simulink model "Attitude"  (R2023b)
settings: Solver=VariableStepAuto  StartTime=0.0  StopTime=10.0  RelTol=1e-3
libraries: simulink_extras x6, aerolibutil x6, vrlib x4, simulink x4, sharedtransform x3, dspindex x3
settings Model: Creator=Saif Mohamed  LastModifiedBy=saifg

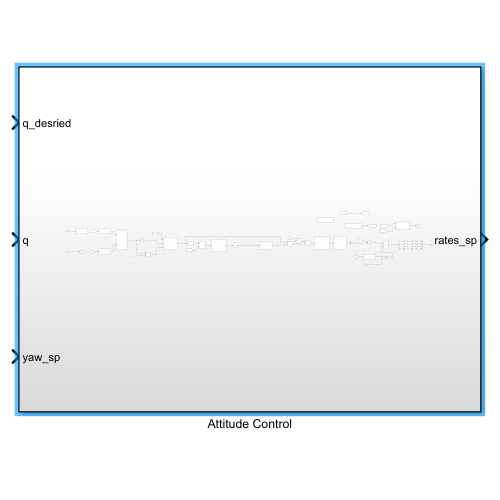
[thumbnail: Simulink's stored preview of the top-level diagram]
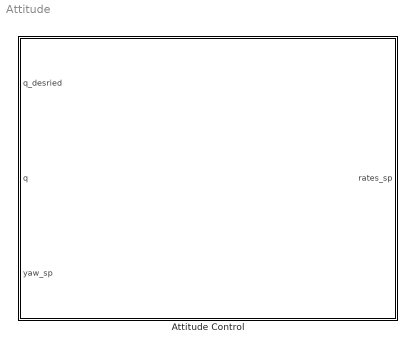
== system Attitude ==
  Attitude Control : Subsystem

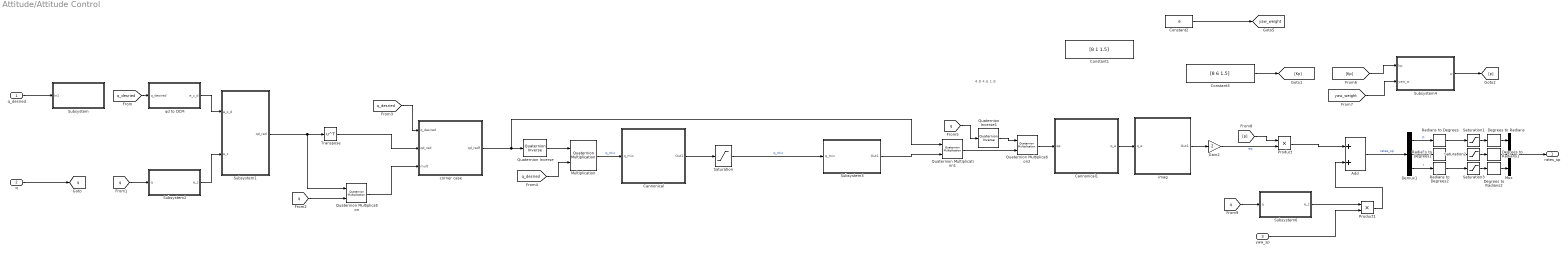
== system Attitude/Attitude Control ==
  note: 4.8 4.6 1.8
  q_desried : Inport
  q : Inport  Port=2
  yaw_sp : Inport  Port=3
  Add : Sum
  Cannonical : Subsystem
  Cannonical1 : Subsystem
  Constant1 : Constant  Value=[8 1 1.5]
  Constant2 : Constant  Value=.6
  Constant3 : Constant  Value=[8 6 1.5]
  Degrees to Radians : simulink_extras/Transformations/Degrees to Radians
  Degrees to Radians1 : simulink_extras/Transformations/Degrees to Radians
  Degrees to Radians2 : simulink_extras/Transformations/Degrees to Radians
  Demux1 : Demux  Outputs=3
  Gain2 : Gain  Gain=2
  Multiplication : aerolibutil/Quaternion Multiplication
  Mux : Mux  Inputs=3
  Product : Product
  Product1 : Product
  Quaternion Inverse : aerolibutil/Quaternion Inverse
  Quaternion Inverse1 : aerolibutil/Quaternion Inverse
  Quaternion Multiplication : aerolibutil/Quaternion Multiplication
  Quaternion Multiplication1 : aerolibutil/Quaternion Multiplication
  Quaternion Multiplication2 : aerolibutil/Quaternion Multiplication
  Radians to Degrees : simulink_extras/Transformations/Radians to Degrees
  Radians to Degrees1 : simulink_extras/Transformations/Radians to Degrees
  Radians to Degrees2 : simulink_extras/Transformations/Radians to Degrees
  Saturation : Saturate  UpperLimit=1  LowerLimit=-1
  Saturation1 : Saturate  UpperLimit=220  LowerLimit=-220
  Saturation2 : Saturate  UpperLimit=220  LowerLimit=-220
  Saturation3 : Saturate  UpperLimit=200  LowerLimit=-200
  Subsystem : Subsystem
  Subsystem1 : Subsystem
  Subsystem2 : Subsystem
  Subsystem3 : Subsystem
  Subsystem4 : Subsystem
  Subsystem6 : Subsystem
  Transpose : Math  Operator=transpose
  corner case : Subsystem
  imag : Subsystem
  qd to DCM : Subsystem
  rates_sp : Outport
  tag scope: q=global, yaw_weight=global
  wires:
  q_desried/1 -> Subsystem/1(In1)
  q/1 -> [q]
  [q_desried] -> qd to DCM/1(q_desired)
  [q] -> Subsystem2/1(q)
  qd to DCM/1(e_z_d) -> Subsystem1/1(e_z_d)
  Subsystem2/1(e_z) -> Subsystem1/2(e_z)
  Subsystem1/1(qd_red) -> Transpose/1, Quaternion Multiplication/1
  [q] -> Quaternion Multiplication/2
  Transpose/1 -> corner case/2(qd_red)
  Quaternion Multiplication/1 -> corner case/3(mult)
  [q_desried] -> corner case/1(q_desired)
  Quaternion Inverse/1 -> Multiplication/1
  [q_desried] -> Multiplication/2
  Multiplication/1 -> Cannonical/1("q_mix ")  "q_mix"
  Cannonical/1(Out1) -> Saturation/1
  Constant2/1 -> [yaw_weight]
  Saturation/1 -> Subsystem3/1(q_mix)  "q_mix"
  Subsystem3/1(Out1) -> Quaternion Multiplication1/2
  Quaternion Multiplication1/1 -> Quaternion Multiplication2/2
  Quaternion Inverse1/1 -> Quaternion Multiplication2/1
  [q] -> Quaternion Inverse1/1
  Quaternion Multiplication2/1 -> Cannonical1/1("qe ")
  Cannonical1/1(q_e) -> imag/1(q_e)
  imag/1(Out1) -> Gain2/1
  Gain2/1 -> Product/2  "eq"
  Constant3/1 -> [Kp]
  [Kp] -> Subsystem4/1(kp)
  [yaw_weight] -> Subsystem4/2(yaw_w)
  Subsystem4/1(p) -> [p]
  [p] -> Product/1
  Product/1 -> Add/1
  [q] -> Subsystem6/1(q)
  Subsystem6/1(e_z) -> Product1/1
  yaw_sp/1 -> Product1/2
  Product1/1 -> Add/2
  Add/1 -> Demux1/1  "rates_sp"
  Demux1/1 -> Radians to Degrees/1  "p"
  Demux1/2 -> Radians to Degrees1/1  "q"
  Demux1/3 -> Radians to Degrees2/1  "r"
  Radians to Degrees/1 -> Saturation1/1
  Radians to Degrees1/1 -> Saturation2/1
  Radians to Degrees2/1 -> Saturation3/1
  Saturation1/1 -> Degrees to Radians/1
  Saturation2/1 -> Degrees to Radians1/1
  Saturation3/1 -> Degrees to Radians2/1
  Mux/1 -> rates_sp/1
  Degrees to Radians/1 -> Mux/1
  Degrees to Radians1/1 -> Mux/2
  Degrees to Radians2/1 -> Mux/3
  corner case/1(qd_redf) -> Quaternion Multiplication1/1, Quaternion Inverse/1

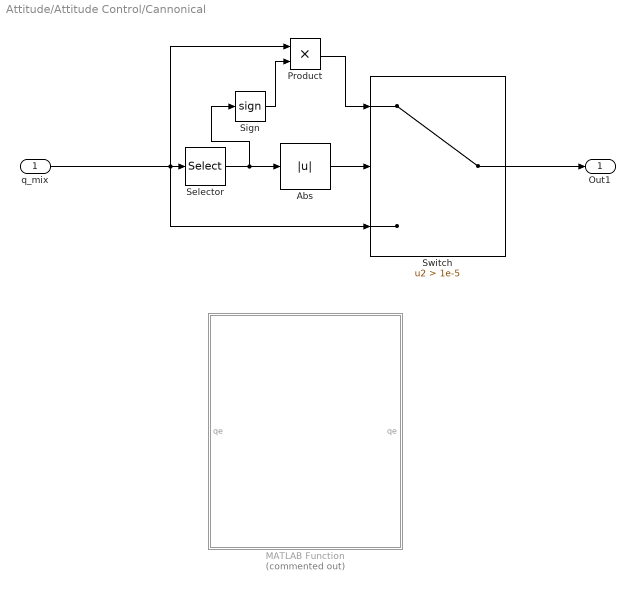
== system Attitude/Attitude Control/Cannonical ==
  "q_mix " : Inport
  Abs : Abs  SaturateOnIntegerOverflow=off
  MATLAB Function : MATLAB Function  Commented=on  TreatAsAtomicUnit=on
  Product : Product
  Selector : Selector  InputPortWidth=4  IndexOptions=Index vector (dialog)  Indices=[1]  OutputSizes=1
  Sign : Signum
  Switch : Switch  Criteria=u2 > Threshold  Threshold=1e-5  SaturateOnIntegerOverflow=off  InputSameDT=off
  Out1 : Outport
  wires:
  "q_mix "/1 -> Product/1, Selector/1, Switch/3
  Selector/1 -> Sign/1, Abs/1
  Abs/1 -> Switch/2
  Switch/1 -> Out1/1
  Product/1 -> Switch/1
  Sign/1 -> Product/2

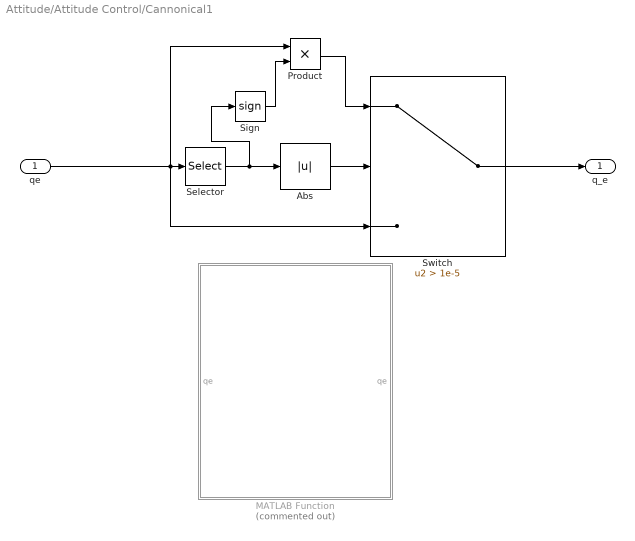
== system Attitude/Attitude Control/Cannonical1 ==
  "qe " : Inport
  Abs : Abs  SaturateOnIntegerOverflow=off
  MATLAB Function : MATLAB Function  Commented=on  TreatAsAtomicUnit=on
  Product : Product
  Selector : Selector  InputPortWidth=4  IndexOptions=Index vector (dialog)  Indices=[1]  OutputSizes=1
  Sign : Signum
  Switch : Switch  Criteria=u2 > Threshold  Threshold=1e-5  SaturateOnIntegerOverflow=off  InputSameDT=off
  q_e : Outport
  wires:
  "qe "/1 -> Product/1, Selector/1, Switch/3
  Selector/1 -> Sign/1, Abs/1
  Abs/1 -> Switch/2
  Switch/1 -> q_e/1
  Product/1 -> Switch/1
  Sign/1 -> Product/2

== system Attitude/Attitude Control/Subsystem ==
  In1 : Inport
  Normalize Vector : vrlib/Utilities/Normalize Vector  maxzero=0
  tag scope: q_desried=global
  wires:
  Normalize Vector/1 -> [q_desried]
  In1/1 -> Normalize Vector/1

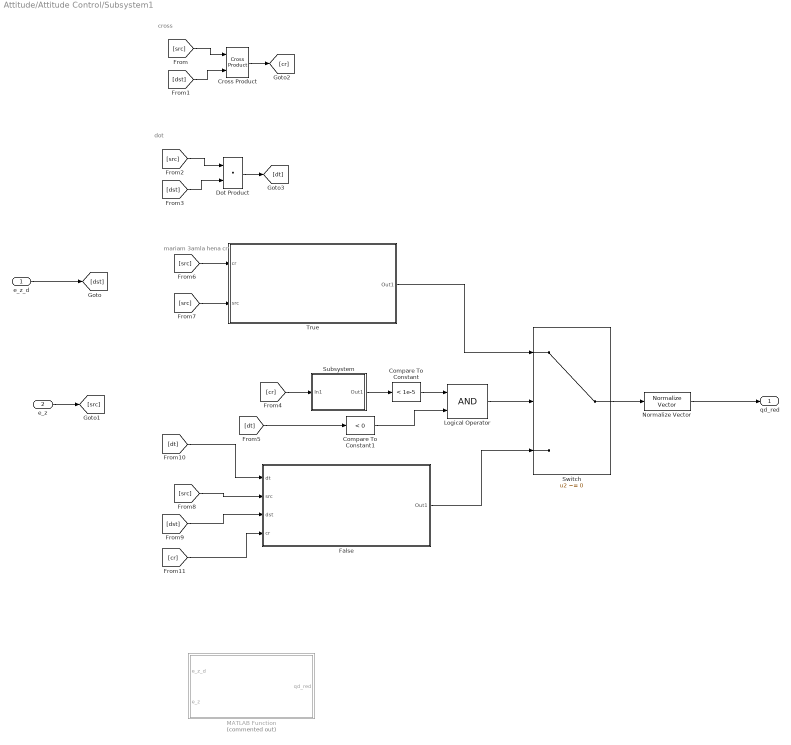
== system Attitude/Attitude Control/Subsystem1 ==
  note: mariam 3amla hena cr
  note: cross
  note: dot
  e_z_d : Inport
  e_z : Inport  Port=2
  Compare To Constant : simulink/Logic and Bit Operations/Compare To Constant  relop=<  const=1e-5  OutDataTypeStr=boolean
  Compare To Constant1 : simulink/Logic and Bit Operations/Compare To Constant  relop=<  const=0  OutDataTypeStr=boolean
  Cross Product : vrlib/Utilities/Cross Product
  Dot Product : DotProduct  OutDataTypeStr=Inherit: Inherit via internal rule
  False : Subsystem
  Logical Operator : Logic  AllPortsSameDT=off  OutDataTypeStr=boolean
  MATLAB Function : MATLAB Function  Commented=on  TreatAsAtomicUnit=on
  Normalize Vector : vrlib/Utilities/Normalize Vector  maxzero=0
  Subsystem : Subsystem
  Switch : Switch  Criteria=u2 ~= 0  SaturateOnIntegerOverflow=off  InputSameDT=off
  True : Subsystem
  qd_red : Outport
  wires:
  e_z_d/1 -> [dst]
  e_z/1 -> [src]
  [src] -> Cross Product/1
  [dst] -> Cross Product/2
  Cross Product/1 -> [cr]
  [src] -> Dot Product/1
  [dst] -> Dot Product/2
  Dot Product/1 -> [dt]
  [cr] -> Subsystem/1(In1)
  Subsystem/1(Out1) -> Compare To Constant/1
  Compare To Constant/1 -> Logical Operator/1
  [dt] -> Compare To Constant1/1
  Compare To Constant1/1 -> Logical Operator/2
  Logical Operator/1 -> Switch/2
  [src] -> True/1(cr)
  [src] -> True/2(src)
  True/1(Out1) -> Switch/1
  [src] -> False/2(src)
  [dst] -> False/3(dst)
  [dt] -> False/1(dt)
  [cr] -> False/4(cr)
  False/1(Out1) -> Switch/3
  Switch/1 -> Normalize Vector/1
  Normalize Vector/1 -> qd_red/1

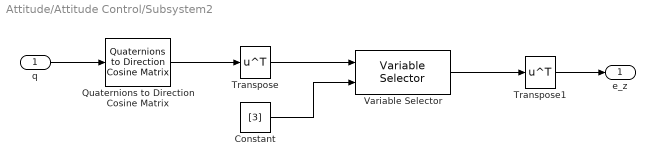
== system Attitude/Attitude Control/Subsystem2 ==
  q : Inport
  Constant : Constant  Value=[3]
  Quaternions to Direction Cosine Matrix : sharedtransform/Quaternions to  Direction Cosine Matrix  aMode=aMode
      settings: LibrarySourceBlock=|
      | aerolibtransform2/Quaternions to
      | Direction Cosine Matrix
  Transpose : Math  Operator=transpose
  Transpose1 : Math  Operator=transpose
  Variable Selector : dspindex/Variable Selector  NumInputs=1  rowsOrCols=Columns  IdxMode=Variable  Elements=[1 3]  ZerOneIdxMode=One-based  errmode=Clip Index  FillMode=on  FillValues=0
  e_z : Outport
  wires:
  Transpose1/1 -> e_z/1
  Variable Selector/1 -> Transpose1/1
  Constant/1 -> Variable Selector/2
  Transpose/1 -> Variable Selector/1
  Quaternions to Direction Cosine Matrix/1 -> Transpose/1
  q/1 -> Quaternions to Direction Cosine Matrix/1

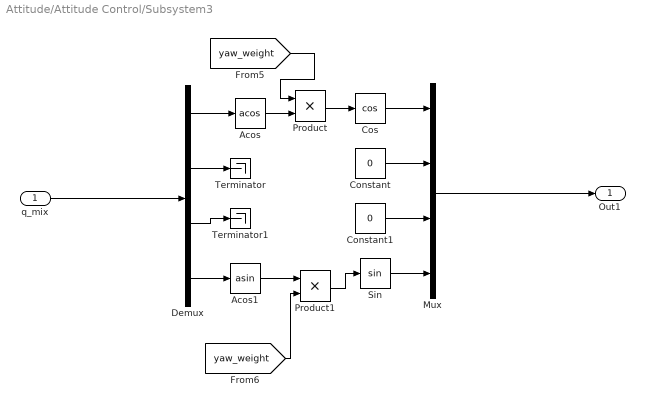
== system Attitude/Attitude Control/Subsystem3 ==
  q_mix : Inport
  Acos : Trigonometry  Operator=acos
  Acos1 : Trigonometry  Operator=asin
  Constant : Constant  Value=0
  Constant1 : Constant  Value=0
  Cos : Trigonometry  Operator=cos
  Demux : Demux
  Mux : Mux
  Product : Product
  Product1 : Product
  Sin : Trigonometry
  Terminator : Terminator
  Terminator1 : Terminator
  Out1 : Outport
  wires:
  Sin/1 -> Mux/4
  Acos/1 -> Product/2
  [yaw_weight] -> Product/1
  Product/1 -> Cos/1
  q_mix/1 -> Demux/1
  Demux/4 -> Acos1/1
  Product1/1 -> Sin/1
  Demux/1 -> Acos/1
  Cos/1 -> Mux/1
  Mux/1 -> Out1/1
  Acos1/1 -> Product1/1
  [yaw_weight] -> Product1/2
  Demux/2 -> Terminator/1
  Demux/3 -> Terminator1/1
  Constant1/1 -> Mux/3
  Constant/1 -> Mux/2

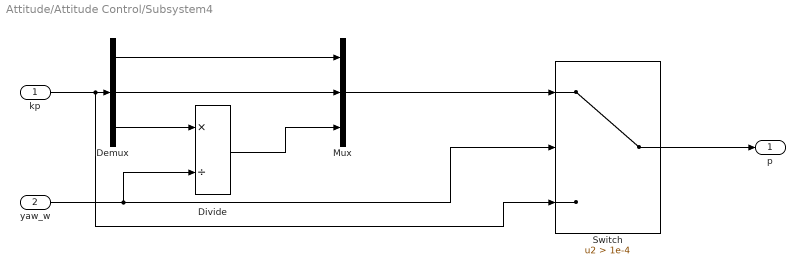
== system Attitude/Attitude Control/Subsystem4 ==
  kp : Inport
  yaw_w : Inport  Port=2
  Demux : Demux  Outputs=3
  Divide : Product  Inputs=*/
  Mux : Mux  Inputs=3
  Switch : Switch  Criteria=u2 > Threshold  Threshold=1e-4  SaturateOnIntegerOverflow=off  InputSameDT=off
  p : Outport
  wires:
  yaw_w/1 -> Switch/2, Divide/2
  Mux/1 -> Switch/1
  kp/1 -> Switch/3, Demux/1
  Demux/1 -> Mux/1
  Demux/2 -> Mux/2
  Demux/3 -> Divide/1
  Divide/1 -> Mux/3
  Switch/1 -> p/1

== system Attitude/Attitude Control/Subsystem6 ==
  q : Inport
  Constant : Constant  Value=[3]
  Quaternions to Direction Cosine Matrix : sharedtransform/Quaternions to  Direction Cosine Matrix  aMode=aMode
      settings: LibrarySourceBlock=|
      | aerolibtransform2/Quaternions to
      | Direction Cosine Matrix
  Transpose : Math  Operator=transpose
  Variable Selector : dspindex/Variable Selector  NumInputs=1  rowsOrCols=Columns  IdxMode=Variable  Elements=[1 3]  ZerOneIdxMode=One-based  errmode=Clip Index  FillMode=on  FillValues=0
  e_z : Outport
  wires:
  Variable Selector/1 -> e_z/1
  Constant/1 -> Variable Selector/2
  Transpose/1 -> Variable Selector/1
  Quaternions to Direction Cosine Matrix/1 -> Transpose/1
  q/1 -> Quaternions to Direction Cosine Matrix/1

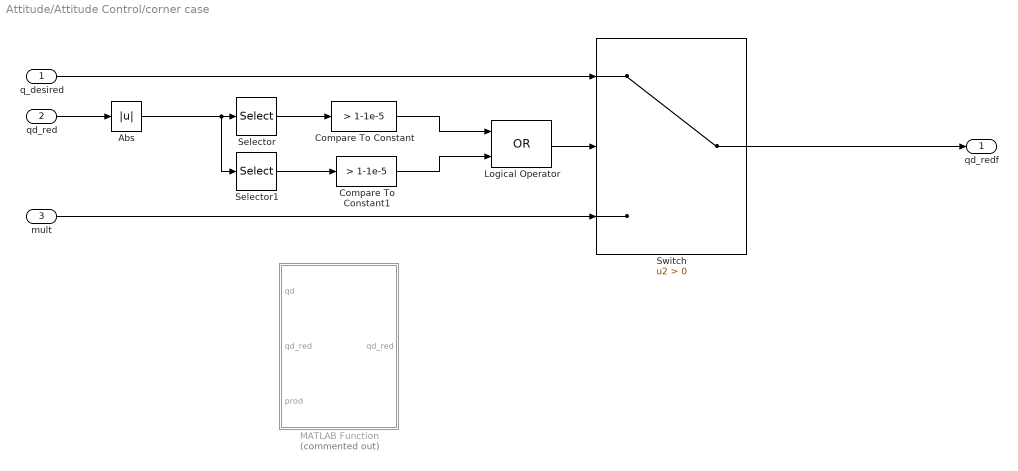
== system Attitude/Attitude Control/corner case ==
  q_desired : Inport
  qd_red : Inport  Port=2
  mult : Inport  Port=3
  Abs : Abs  SaturateOnIntegerOverflow=off
  Compare To Constant : simulink/Logic and Bit Operations/Compare To Constant  relop=>  const=1-1e-5  OutDataTypeStr=boolean
  Compare To Constant1 : simulink/Logic and Bit Operations/Compare To Constant  relop=>  const=1-1e-5  OutDataTypeStr=boolean
  Logical Operator : Logic  Operator=OR  AllPortsSameDT=off  OutDataTypeStr=boolean
  MATLAB Function : MATLAB Function  Commented=on  TreatAsAtomicUnit=on
  Selector : Selector  InputPortWidth=4  IndexOptions=Index vector (dialog)  Indices=[2]  OutputSizes=1
  Selector1 : Selector  InputPortWidth=4  IndexOptions=Index vector (dialog)  Indices=[3]  OutputSizes=1
  Switch : Switch  Criteria=u2 > Threshold  SaturateOnIntegerOverflow=off  InputSameDT=off
  qd_redf : Outport
  wires:
  Abs/1 -> Selector1/1, Selector/1
  Selector/1 -> Compare To Constant/1
  Selector1/1 -> Compare To Constant1/1
  Compare To Constant/1 -> Logical Operator/1
  Compare To Constant1/1 -> Logical Operator/2
  Switch/1 -> qd_redf/1
  Logical Operator/1 -> Switch/2
  q_desired/1 -> Switch/1
  mult/1 -> Switch/3
  qd_red/1 -> Abs/1

== system Attitude/Attitude Control/imag ==
  q_e : Inport
  Demux : Demux
  Mux : Mux  Inputs=3
  Terminator : Terminator
  Out1 : Outport
  wires:
  Mux/1 -> Out1/1
  q_e/1 -> Demux/1
  Demux/1 -> Terminator/1
  Demux/2 -> Mux/1
  Demux/3 -> Mux/2
  Demux/4 -> Mux/3

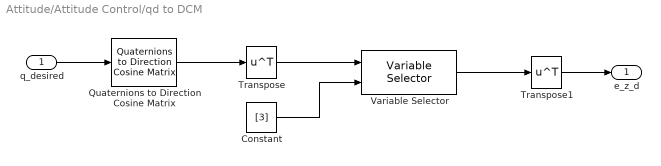
== system Attitude/Attitude Control/qd to DCM ==
  q_desired : Inport
  Constant : Constant  Value=[3]
  Quaternions to Direction Cosine Matrix : sharedtransform/Quaternions to  Direction Cosine Matrix  aMode=aMode
      settings: LibrarySourceBlock=|
      | aerolibtransform2/Quaternions to
      | Direction Cosine Matrix
  Transpose : Math  Operator=transpose
  Transpose1 : Math  Operator=transpose
  Variable Selector : dspindex/Variable Selector  NumInputs=1  rowsOrCols=Columns  IdxMode=Variable  Elements=[1 3]  ZerOneIdxMode=One-based  errmode=Clip Index  FillMode=on  FillValues=0
  e_z_d : Outport
  wires:
  q_desired/1 -> Quaternions to Direction Cosine Matrix/1
  Quaternions to Direction Cosine Matrix/1 -> Transpose/1
  Transpose/1 -> Variable Selector/1
  Constant/1 -> Variable Selector/2
  Variable Selector/1 -> Transpose1/1
  Transpose1/1 -> e_z_d/1

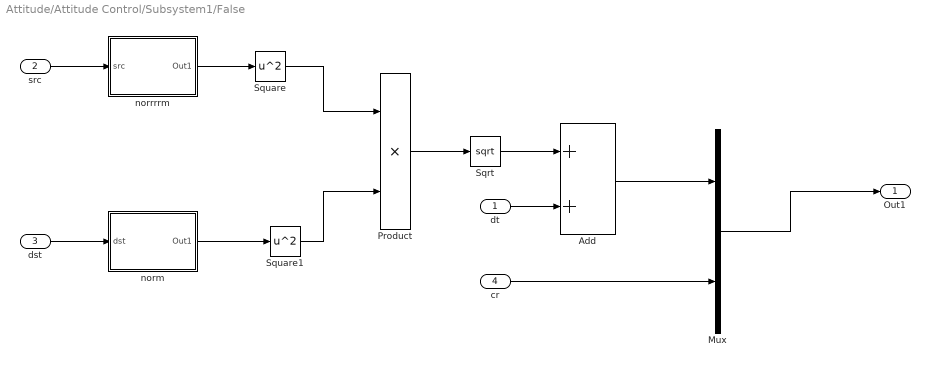
== system Attitude/Attitude Control/Subsystem1/False ==
  dt : Inport
  src : Inport  Port=2
  dst : Inport  Port=3
  cr : Inport  Port=4
  Add : Sum
  Mux : Mux  Inputs=2
  Product : Product
  Sqrt : Sqrt
  Square : Math  Operator=square
  Square1 : Math  Operator=square
  norm : Subsystem
  norrrrm : Subsystem
  Out1 : Outport
  wires:
  src/1 -> norrrrm/1(src)
  dst/1 -> norm/1(dst)
  norrrrm/1(Out1) -> Square/1
  norm/1(Out1) -> Square1/1
  Square/1 -> Product/1
  Square1/1 -> Product/2
  Product/1 -> Sqrt/1
  Sqrt/1 -> Add/1
  dt/1 -> Add/2
  Add/1 -> Mux/1
  Mux/1 -> Out1/1
  cr/1 -> Mux/2

== system Attitude/Attitude Control/Subsystem1/Subsystem ==
  In1 : Inport
  Square : Math  Operator=square
  Square1 : Math  Operator=square
  Sum of Elements : Sum  Inputs=+
  Out1 : Outport
  wires:
  In1/1 -> Square/1
  Square/1 -> Sum of Elements/1
  Sum of Elements/1 -> Square1/1
  Square1/1 -> Out1/1

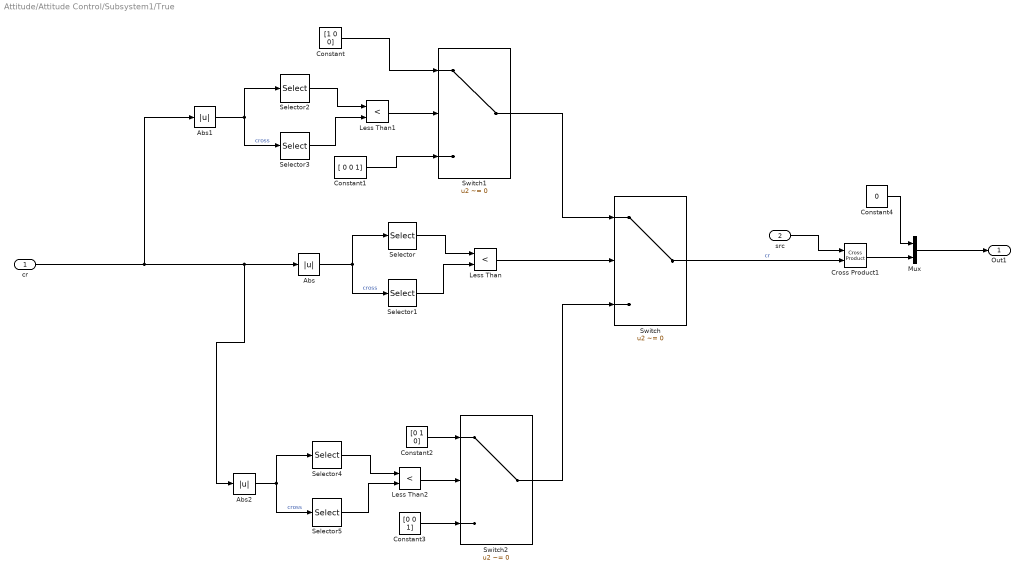
== system Attitude/Attitude Control/Subsystem1/True ==
  cr : Inport
  src : Inport  Port=2
  Abs : Abs  SaturateOnIntegerOverflow=off
  Abs1 : Abs  SaturateOnIntegerOverflow=off
  Abs2 : Abs  SaturateOnIntegerOverflow=off
  Constant : Constant  Value=[1 0 0]
  Constant1 : Constant  Value=[ 0 0 1]
  Constant2 : Constant  Value=[0 1 0]
  Constant3 : Constant  Value=[0 0 1]
  Constant4 : Constant  Value=0
  Cross Product1 : vrlib/Utilities/Cross Product
  Less Than : RelationalOperator  Operator=<  OutDataTypeStr=boolean  RndMeth=Simplest  InputSameDT=off
  Less Than1 : RelationalOperator  Operator=<  OutDataTypeStr=boolean  RndMeth=Simplest  InputSameDT=off
  Less Than2 : RelationalOperator  Operator=<  OutDataTypeStr=boolean  RndMeth=Simplest  InputSameDT=off
  Mux : Mux  Inputs=2
  Selector : Selector  InputPortWidth=3  IndexOptions=Index vector (dialog)  Indices=[1]  OutputSizes=1
  Selector1 : Selector  InputPortWidth=3  IndexOptions=Index vector (dialog)  Indices=[2]  OutputSizes=1
  Selector2 : Selector  InputPortWidth=3  IndexOptions=Index vector (dialog)  Indices=[1]  OutputSizes=1
  Selector3 : Selector  InputPortWidth=3  IndexOptions=Index vector (dialog)  Indices=[3]  OutputSizes=1
  Selector4 : Selector  InputPortWidth=3  IndexOptions=Index vector (dialog)  Indices=[2]  OutputSizes=1
  Selector5 : Selector  InputPortWidth=3  IndexOptions=Index vector (dialog)  Indices=[3]  OutputSizes=1
  Switch : Switch  Criteria=u2 ~= 0  SaturateOnIntegerOverflow=off  InputSameDT=off
  Switch1 : Switch  Criteria=u2 ~= 0  SaturateOnIntegerOverflow=off  InputSameDT=off
  Switch2 : Switch  Criteria=u2 ~= 0  SaturateOnIntegerOverflow=off  InputSameDT=off
  Out1 : Outport
  wires:
  Selector/1 -> Less Than/1
  Selector1/1 -> Less Than/2
  Less Than/1 -> Switch/2
  Switch1/1 -> Switch/1
  Selector3/1 -> Less Than1/2
  Selector2/1 -> Less Than1/1
  cr/1 -> Abs2/1, Abs/1, Abs1/1
  Less Than1/1 -> Switch1/2
  Abs/1 -> Selector1/1, Selector/1  "cross"
  Abs1/1 -> Selector3/1, Selector2/1  "cross"
  Constant/1 -> Switch1/1
  Constant1/1 -> Switch1/3
  Switch2/1 -> Switch/3
  Selector5/1 -> Less Than2/2
  Less Than2/1 -> Switch2/2
  Selector4/1 -> Less Than2/1
  Abs2/1 -> Selector5/1, Selector4/1  "cross"
  Constant2/1 -> Switch2/1
  Constant3/1 -> Switch2/3
  Switch/1 -> Cross Product1/2  "cr"
  src/1 -> Cross Product1/1
  Cross Product1/1 -> Mux/2
  Constant4/1 -> Mux/1
  Mux/1 -> Out1/1

== system Attitude/Attitude Control/Subsystem1/False/norm ==
  dst : Inport
  Square : Math  Operator=square
  Square1 : Math  Operator=square
  Sum of Elements : Sum  Inputs=+
  Out1 : Outport
  wires:
  Square1/1 -> Out1/1
  Sum of Elements/1 -> Square1/1
  Square/1 -> Sum of Elements/1
  dst/1 -> Square/1

== system Attitude/Attitude Control/Subsystem1/False/norrrrm ==
  src : Inport
  Square : Math  Operator=square
  Square1 : Math  Operator=square
  Sum of Elements : Sum  Inputs=+
  Out1 : Outport
  wires:
  src/1 -> Square/1
  Square/1 -> Sum of Elements/1
  Sum of Elements/1 -> Square1/1
  Square1/1 -> Out1/1

== matlab function Attitude/Attitude Control/Cannonical/MATLAB Function ==
  data: qe input; qe output
function qe = fcn(qe)

    if abs(qe(1)) > 1e-5
        qe=qe*sign(qe(1));
    end
end

== matlab function Attitude/Attitude Control/Subsystem1/MATLAB Function ==
  data: qd_red output; e_z_d input; e_z input
function qd_red = fcn(e_z_d, e_z)
qd_red=[0 0 0 0];
src=e_z;
dst=e_z_d;
eps=1e-5;

cr=cross(src,dst);
dt=dot(src,dst);

if norm(cr) < eps && dt<0
    cr=abs(src);

    if (cr(1) < cr(2))
        if (cr(1) < cr(3))
            cr=[1 0 0];
        else
            cr=[0 0 1];
        end
    else
        if (cr(2) < cr(3))
            cr=[0 1 0];
        else
            cr=[0 0 1];
        end
    end
    qd_red(1)=0;
    cr=cross(src,cr);
else
    qd_red(1)=dt+sqrt((norm(src)^2) * (norm(dst))^2);
end
qd_red(2)=cr(1);
qd_red(3)=cr(2);
qd_red(4)=cr(3);

qd_red=qd_red/norm(qd_red);        
end

== matlab function Attitude/Attitude Control/corner case/MATLAB Function ==
  data: qd input; qd_red input; qd_red output; prod input
function qd_red = fcn(qd, qd_red,prod)

if abs(qd_red(2)) > (1-1e-5) || abs(qd_red(3)) > (1-1e-5)
    qd_red=qd;
else
    qd_red=prod;
    
end

== matlab function Attitude/Attitude Control/Cannonical1/MATLAB Function ==
  data: qe input; qe output
function qe = fcn(qe)

    if abs(qe(1)) > 1e-5
        qe=qe*sign(qe(1));
    end
end
